simulink model "ball_beam"  (R2017b)
settings: Solver=VariableStepAuto  StartTime=0.0  StopTime=10.0  RelTol=1e-3
libraries: fuzblock x1
settings Model: Creator=dhruvlaad  LastModifiedBy=dhruvlaad

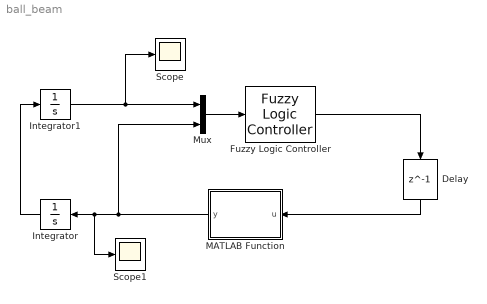
== system ball_beam ==
  Delay : Delay  DelayLength=1  InitialCondition=0
  Fuzzy Logic Controller : fuzblock/Fuzzy Logic  Controller  FIS='ball_beam.fis'  OutputSampleNumber=101  DataType=double  FuzzifiedInputs=off  RuleFiringStrengths=off  RuleOutputs=off  AggregatedOutputs=off  SimulateUsing=Interpreted execution
  Integrator : Integrator
  Integrator1 : Integrator  InitialCondition=0.25
  MATLAB Function : MATLAB Function  TreatAsAtomicUnit=on
  Mux : Mux  Inputs=2
  Scope : Scope
  Scope1 : Scope
  wires:
  Fuzzy Logic Controller/1 -> Delay/1
  Integrator/1 -> Integrator1/1
  Mux/1 -> Fuzzy Logic Controller/1
  Integrator1/1 -> Scope/1, Mux/1
  MATLAB Function/1(y) -> Mux/2, Scope1/1, Integrator/1
  Delay/1 -> MATLAB Function/1(u)

== matlab function ball_beam/MATLAB Function ==
  data: u input; y output
function y = fcn(u)

y = 9.81*sin(0.2*u);
